simulink model "TrustAI_merge"  (R2023b)
settings: Solver=FixedStepAuto  StartTime=0.0  StopTime=10.0  RelTol=1e-3
libraries: robotlib x4
settings Model: Creator=yuweiyang  LastModifiedBy=yuweiyang
settings OptimizationCC: EnhancedBackFolding=on  PassReuseOutputArgsAs=Individual arguments  ZeroExternalMemoryAtStartup=off  ZeroInternalMemoryAtStartup=off  MaxStackSize=64  OptimizeBlockOrder=speed  DifferentSizesBufferReuse=on  OptimizationCustomize=off  EfficientTunableParamExpr=on
settings DebuggingCC: ParameterTunabilityLossMsg=error
settings HardwareCC: ProdBitPerPointer=32  ProdBitPerSizeT=32  ProdBitPerPtrDiffT=32  ProdLargestAtomicFloat=None  ProdIntDivRoundTo=Undefined  ProdEndianess=Unspecified  ProdWordSize=32  ProdHWDeviceType=Generic->Unspecified (assume 32-bit Generic)
settings SFSimCC: MATLABDynamicMemAlloc=off
settings RTWCC: Description=Embedded Coder  SystemTargetFile=ert.tlc  HardwareBoard=Robot Operating System (ROS)  TLCOptions="-aInlineSetEventsForThisBaseRateFcn=TLC_FALSE -aSuppressMultiTaskScheduler=TLC_FALSE  -aRateBasedStepFcn=0"  GenCodeOnly=on  TemplateMakefile=ert_default_tmf  Toolchain=Catkin  TargetLang=C++
settings CodeAppCC: ForceParamTrailComments=on  IgnoreCustomStorageClasses=off  OperatorAnnotations=on  SimulinkDataObjDesc=on  SFDataObjDesc=on  InsertBlockDesc=on

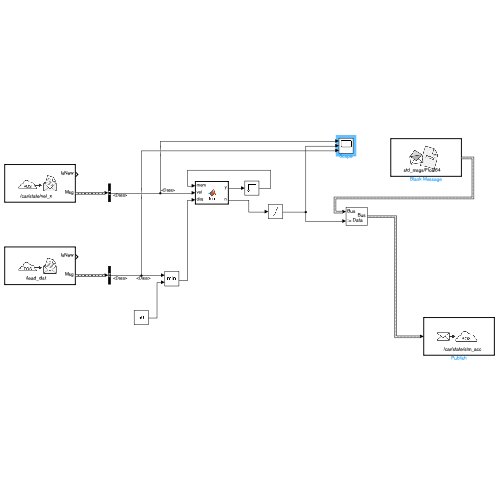
[thumbnail: Simulink's stored preview of the top-level diagram]
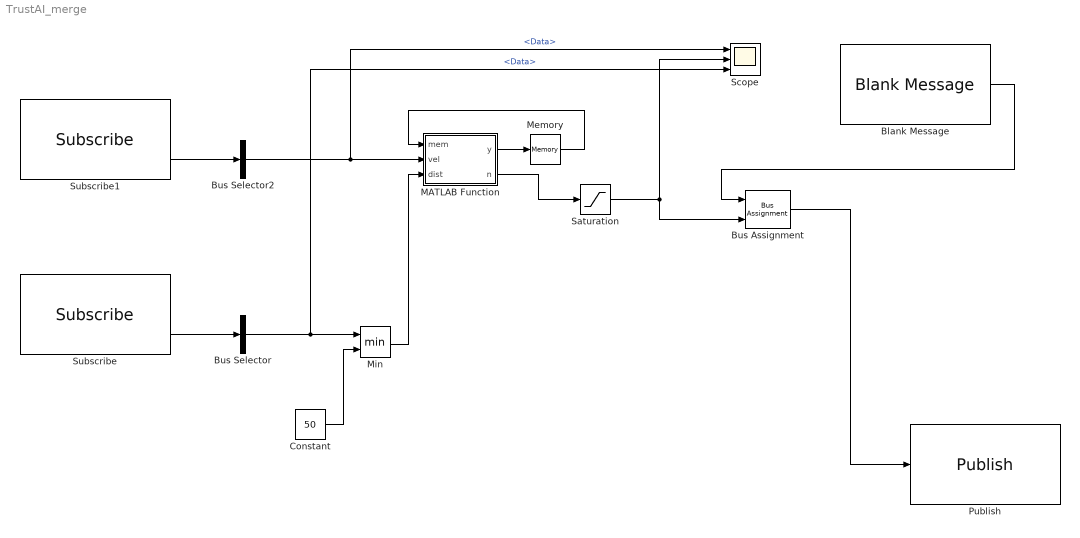
== system TrustAI_merge ==
  Blank Message : robotlib/Blank Message  messageClass=Message  entityType=std_msgs/Float64  messageType=std_msgs/Float64  SampleTime=inf  legacyBusStruct=off
  Bus Assignment : BusAssignment  AssignedSignals=Data
  Bus Selector : BusSelector  OutputSignals=Data
  Bus Selector2 : BusSelector  OutputSignals=Data
  Constant : Constant  Value=50
  MATLAB Function : MATLAB Function  TreatAsAtomicUnit=on
  Memory : Memory  InitialCondition=-1
  Min : MinMax  Inputs=2
  Publish : robotlib/Publish  topicSource=Specify your own  topic=/car/state/sim_acc  messageType=std_msgs/Float64  legacyBusStruct=off  messageQueueLength=1
  Saturation : Saturate
  Scope : Scope  NumInputPorts=3
  Subscribe : robotlib/Subscribe  topicSource=Specify your own  topic=/lead_dist  messageType=std_msgs/Float64  SampleTime=-1  legacyBusStruct=off  messageQueueLength=1
  Subscribe1 : robotlib/Subscribe  topicSource=Specify your own  topic=/car/state/vel_x  messageType=std_msgs/Float64  SampleTime=-1  legacyBusStruct=off  messageQueueLength=1
  wires:
  Subscribe/2 -> Bus Selector/1
  Constant/1 -> Min/2
  Subscribe1/2 -> Bus Selector2/1
  MATLAB Function/1(y) -> Memory/1
  Memory/1 -> MATLAB Function/1(mem)
  Min/1 -> MATLAB Function/3(dist)
  Saturation/1 -> Scope/2, Bus Assignment/2
  MATLAB Function/2(n) -> Saturation/1
  Bus Assignment/1 -> Publish/1
  Bus Selector/1 -> Scope/3, Min/1  "<Data>"
  Bus Selector2/1 -> MATLAB Function/2(vel), Scope/1  "<Data>"
  Blank Message/1 -> Bus Assignment/1

== matlab function TrustAI_merge/MATLAB Function ==
  data: mem input; vel input; dist input; y output; n output
function [y, n] = fcn(mem, vel, dist)
    
    if (mem ~= -1)
        vel_desire = mem;
    else 
        vel_desire = vel * 0.8;
        mem = vel_desire;
    end

    
    k1 = 0.01;
    k2 = 0.3;
    headway = 3;

    n = k1 * (dist - headway * vel) + k2 * (vel_desire - vel);
    y = mem;
end
